simulink model "diabetes_model"  (Simulink 7.9)
settings: Solver=ode45  StartTime=0.0  StopTime=400  MaxStep=1  RelTol=1e-3
values from neighbouring files (symbols this model uses):
  D = 0.05:.05:0.5    [Ch01_Matlab_Tips.m]    (also in Ch04_PredatorPrey.m = jacobian(@(u)g(xss,u),0); Ch08_Bioreactor_Continuous.m = @(t,x) max(0, 0.1 + Kp*(Sp(t) - x(2)) + Ki*x(4)); Ch12_PID.m = Kp*tf([Td 0],[Td/N 1],'TimeUnit','minutes'); Ch12_PID_2DOF.m = @(Td) tf([Td 0],[Td/10 1],'TimeUnit','minutes'))
  Gb = 81    [Ch23_E03_diabetes.m]
  Ib = 15    [Ch23_E03_diabetes.m]
  n = size(idx,1)    [Ch21_DataFitting.m]    (also in Ch23_E03_diabetes.m = 0.0926)
  p1 = 0.028735    [Ch23_E03_diabetes.m]
  p2 = 0.028344    [Ch23_E03_diabetes.m]
  p3 = 5.035e-5    (= 5.035e-05)    [Ch23_E03_diabetes.m]
  U = @(t) 15 + 100*(t <= 8)    [Ch23_E03_diabetes.m]
  V = 4000    [Ch02_BlendingTank.m]    (also in Ch02_Braatz.m = deval(Vsoln,t); Ch02_ClassDemo.m; Ch02_E05_CSTR.m = 100; Ch08_BlendingTankControl.m)
settings Model: Creator=jeff  LastModifiedBy=jeff
settings DebuggingCC: FcnCallInpInsideContextMsg=Use local settings
settings GRTTargetCC: CombineOutputUpdateFcns=off  GRTInterface=on

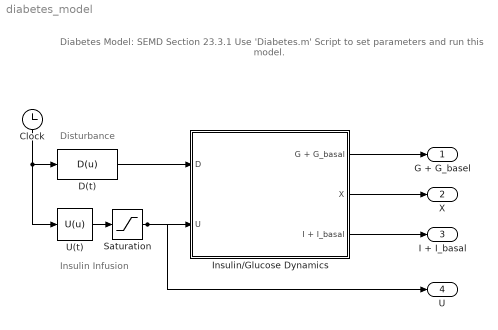
== system diabetes_model ==
  note: Diabetes Model: SEMD Section 23.3.1
      |
      |     Use 'Diabetes.m' Script to set parameters and run this model.
  note: Disturbance
  note: Insulin Infusion
  Clock : Clock
  D(t) : MATLABFcn  MATLABFcn=D(u)
  Insulin/Glucose Dynamics : Subsystem
  Saturation : Saturate  UpperLimit=115  LowerLimit=0
  U(t) : MATLABFcn  MATLABFcn=U(u)
  G + G_basel : Outport
  X : Outport  Port=2
  I + I_basal : Outport  Port=3
  U : Outport  Port=4
  wires:
  U(t)/1 -> Saturation/1
  Saturation/1 -> U/1, Insulin/Glucose Dynamics/2(U)
  Clock/1 -> D(t)/1, U(t)/1
  D(t)/1 -> Insulin/Glucose Dynamics/1(D)
  Insulin/Glucose Dynamics/1(G + G_basal) -> G + G_basel/1
  Insulin/Glucose Dynamics/2(X) -> X/1
  Insulin/Glucose Dynamics/3(I + I_basal) -> I + I_basal/1

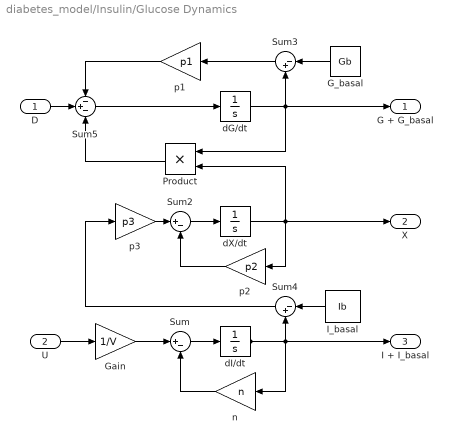
== system diabetes_model/Insulin/Glucose Dynamics ==
  D : Inport
  U : Inport  Port=2
  G_basal : Constant  Value=Gb
  Gain : Gain  Gain=1/V
  I_basal : Constant  Value=Ib
  Product : Product  RndMeth=Zero
  Sum : Sum  Inputs=|+-
  Sum2 : Sum  Inputs=|+-
  Sum3 : Sum  Inputs=|-+
  Sum4 : Sum  Inputs=|-+
  Sum5 : Sum  Inputs=-+-
  dG/dt : Integrator  InitialCondition=81
  dI/dt : Integrator  InitialCondition=Ib
  dX/dt : Integrator
  n : Gain  Gain=n
  p1 : Gain  Gain=p1
  p2 : Gain  Gain=p2
  p3 : Gain  Gain=p3
  G + G_basal : Outport
  X : Outport  Port=2
  I + I_basal : Outport  Port=3
  wires:
  dI/dt/1 -> n/1, I + I_basal/1, Sum4/2
  Gain/1 -> Sum/1
  Sum/1 -> dI/dt/1
  n/1 -> Sum/2
  p3/1 -> Sum2/1
  Sum2/1 -> dX/dt/1
  dX/dt/1 -> p2/1, Product/2, X/1
  p2/1 -> Sum2/2
  dG/dt/1 -> Product/1, Sum3/2, G + G_basal/1
  Sum5/1 -> dG/dt/1
  Product/1 -> Sum5/3
  G_basal/1 -> Sum3/1
  Sum3/1 -> p1/1
  p1/1 -> Sum5/1
  I_basal/1 -> Sum4/1
  Sum4/1 -> p3/1
  U/1 -> Gain/1
  D/1 -> Sum5/2
